simulink model "Vehicle_Model_2Track_OLD"  (R2022b)
settings: Solver=ode2  StartTime=0  StopTime=Tf  FixedStep=Ts  EnableMultiTasking=on
model workspace (MAT data in the model file):
  aKalman = Simulink.Parameter
  aKalman.DataType = 'auto'
  aKalman.Complexity = 'real'
  aKalman.Dimensions = [0 0]
  slipEnabler = Simulink.Parameter
  slipEnabler.DataType = 'auto'
  slipEnabler.Complexity = 'real'
  slipEnabler.Dimensions = [0 0]
values from neighbouring files (symbols this model uses):
  flg = 1    [mainVehicleModel_2Track.m]
  slope = 0.5    [mainVehicleModel_2Track.m]
  steer_des = 10    [mainVehicleModel_2Track.m]
  V_des = 50/3.6    (= 13.8888888889)    [mainVehicleModel_2Track.m]
  X0 = loadInitialConditions(V0)    [mainVehicleModel_2Track.m]
undefined symbols (not defined in the file or in its folder): DiscIntNeverNeededParam
libraries: simulink_extras x12, simulink x2, slpidlib x1
settings Model: Creator=Edoardo  LastModifiedBy=giorg
settings SolverCC: AlgebraicLoopSolver=TrustRegion
settings DataIOCC: LimitDataPoints=on  SaveFormat=StructureWithTime
settings OptimizationCC: BlockReduction=off  DefaultParameterBehavior=Inlined  BufferReuse=off  PassReuseOutputArgsAs=Individual arguments  MaxStackSize=64  EfficientTunableParamExpr=on
settings DebuggingCC: ReadBeforeWriteMsg=DisableAll  WriteAfterWriteMsg=DisableAll  WriteAfterReadMsg=DisableAll  AlgebraicLoopMsg=none  MultiTaskDSMMsg=none  ParameterTunabilityLossMsg=error  PregeneratedLibrarySubsystemCodeDiagnostic=none  SFUnexpectedBacktrackingDiag=warning  SFNoUnconditionalDefaultTransitionDiag=warning  SFExecutionAtInitializationDiag=none  ArithmeticOperatorsInVariantConditions=warning
settings HardwareCC: ProdBitPerInt=16  ProdBitPerPointer=16  ProdBitPerSizeT=16  ProdBitPerPtrDiffT=16  ProdLargestAtomicFloat=None  ProdWordSize=16  ProdHWDeviceType=STMicroelectronics->ST10/Super10
settings ModelReferenceCC: UpdateModelReferenceTargets=IfOutOfDate  EnableRefExpFcnMdlSchedulingChecks=on  PropagateSignalLabelsOutOfModel=off
settings SFSimCC: SFSimEcho=off  SimUseLocalCustomCode=off  MATLABDynamicMemAlloc=off  CustomCodeUndefinedFunction=UseInterfaceOnly
settings RTWCC: Description=Embedded Coder  SystemTargetFile=ert.tlc  TemplateMakefile=ert_default_tmf  GenerateReport=on  RetainRTWFile=on  RTWUseLocalCustomCode=off  Toolchain=GNU Tools for ARM Embedded Processors  BuildConfiguration=Faster Runs  IncludeHyperlinkInReport=on  LaunchReport=on  GenerateTraceInfo=on  GenerateTraceReport=on  GenerateTraceReportSl=on  GenerateTraceReportSf=on  GenerateTraceReportEml=on  DLArmComputeVersion=19.05
settings CodeAppCC: ForceParamTrailComments=on  IgnoreCustomStorageClasses=off  OperatorAnnotations=on  SimulinkDataObjDesc=on  SFDataObjDesc=on  InsertBlockDesc=on
settings ERTTargetCC: CodeReplacementLibrary=ARM Cortex-M (Optimized)  SupportVariableSizeSignals=on  RootIOFormat=Structure reference  ERTCustomFileTemplate=example_file_process.tlc
settings ConfigComp: CovMetricSettings=dw  CovSaveCumulativeToWorkspaceVar=on  CovSaveSingleToWorkspaceVar=on  CovExternalEMLEnable=off
settings ExplorerConfigSet: SimMechanicsOpenEditorOnUpdate=off

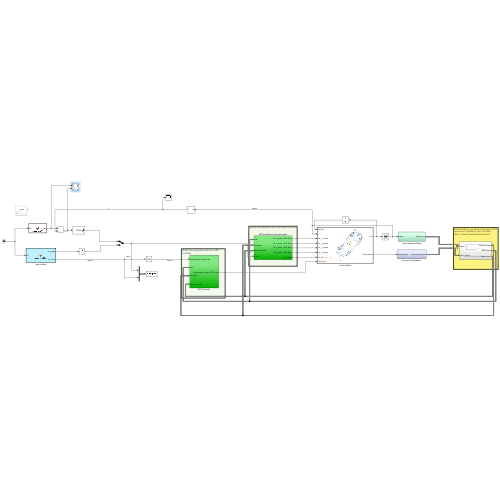
[thumbnail: Simulink's stored preview of the top-level diagram]
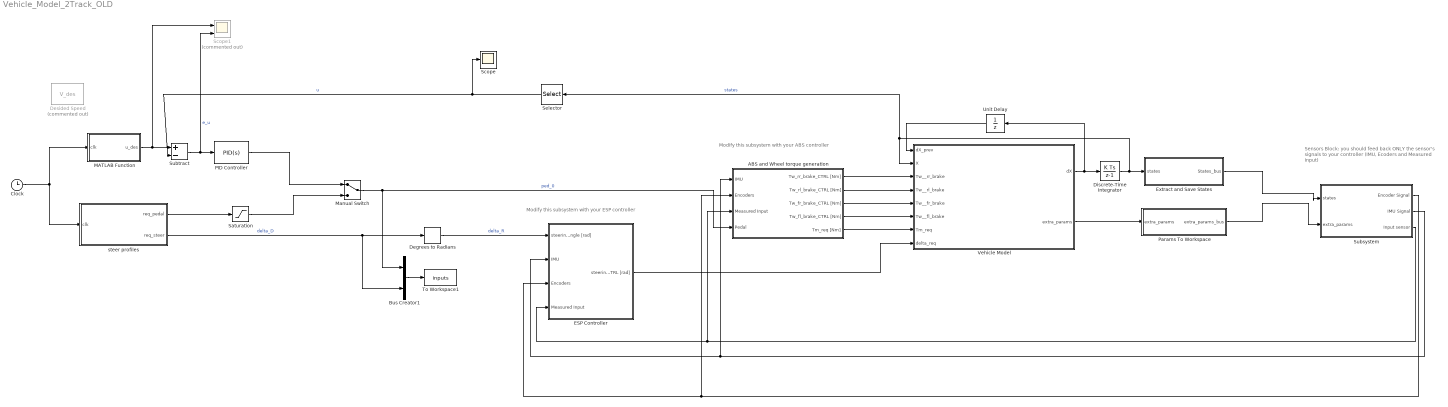
== system Vehicle_Model_2Track_OLD ==
  note: Modify this subsystem with your ESP
      | controller
  note: Modify this subsystem with your ABS controller
  note: Sensors Block: you should feed back ONLY
      | the sensor's signals to your controller
      | (IMU, Ecoders and Measured Input)
  ABS and Wheel torque generation : Subsystem
  Bus Creator1 : BusCreator  Inputs=2
  Clock : Clock
  Degrees to Radians : simulink_extras/Transformations/Degrees to Radians
  Desided Speed : Constant  Commented=on  Value=V_des
  Discrete-Time Integrator : DiscreteIntegrator  gainval=1  InitialCondition=X0  SampleTime=-1  ICPrevOutput=DiscIntNeverNeededParam  ICPrevScaledInput=DiscIntNeverNeededParam
  ESP Controller : Subsystem
  Extract and Save States : Subsystem
  MATLAB Function : MATLAB Function  TreatAsAtomicUnit=on
  Manual Switch : ManualSwitch
  PID Controller : slpidlib/PID Controller  Controller=PID  Form=Parallel  TimeDomain=Continuous-time  UseExternalTs=off  SampleTime=-1  IntegratorMethod=Forward Euler  FilterMethod=Forward Euler  ControllerParametersSource=internal  P=0.0436462066049939  I=0.0175035310088279  UseKiTs=off  D=-0.00909870879334459  N=2  UseFilter=on  TunerSelectOption=Transfer Function Based (PID Tuner App)  InitialConditionSource=internal  InitialConditionForIntegrator=0  InitialConditionForFilter=0  DifferentiatorICPrevScaledInput=0  ExternalReset=none  TrackingMode=off  Kt=1  LimitOutput=on  SatLimitsSource=internal  UpperSaturationLimit=1  LowerSaturationLimit=-1  LinearizeAsGain=on  AntiWindupMode=none  Kb=1  LimitIntegrator=off  UpperIntegratorSaturationLimit=inf  LowerIntegratorSaturationLimit=-inf  POutMin=[]  POutMax=[]  IOutMin=[]  IOutMax=[]  DOutMin=[]  DOutMax=[]  NOutMin=[]  NOutMax=[]  SumOutMin=[]  SumOutMax=[]  SaturationOutMin=[]  SaturationOutMax=[]  PParamMin=[]  PParamMax=[]  IParamMin=[]  IParamMax=[]  DParamMin=[]  DParamMax=[]  NParamMin=[]  NParamMax=[]  KbParamMin=[]  KbParamMax=[]  KtParamMin=[]  KtParamMax=[]  KbOutMin=[]  KbOutMax=[]  KtOutMin=[]  KtOutMax=[]  IntegratorOutMin=[]  IntegratorOutMax=[]  FilterOutMin=[]  FilterOutMax=[]  SumI1OutMin=[]  SumI1OutMax=[]  SumI2OutMin=[]  SumI2OutMax=[]  SumI3OutMin=[]  SumI3OutMax=[]  SumI4OutMin=[]  SumI4OutMax=[]  SumDOutMin=[]  SumDOutMax=[]  DifferentiatorOutMin=[]  DifferentiatorOutMax=[]  FilterDiffOutCoefMin=[]  FilterDiffOutCoefMax=[]  ReciprocalOutMin=[]  ReciprocalOutMax=[]  SumDenOutMin=[]  SumDenOutMax=[]  SumNumOutMin=[]  SumNumOutMax=[]  DivideOutMin=[]  DivideOutMax=[]  UdiffTsProdOutMin=[]  UdiffTsProdOutMax=[]  NTsProdOutMin=[]  NTsProdOutMax=[]  UintegralTsProdOutMin=[]  UintegralTsProdOutMax=[]  UngainTsProdOutMin=[]  UngainTsProdOutMax=[]  ClampingZeroOutDataTypeStr=Inherit: Inherit via back propagation  ClampingZeroOutMin=[]  ClampingZeroOutMax=[]  FilterDenConstantOutDataTypeStr=Inherit: Inherit via back propagation  FilterDenConstantOutMin=[]  FilterDenConstantOutMax=[]  PCopyOutDataTypeStr=Inherit: Inherit via back propagation  PCopyOutMin=[]  PCopyOutMax=[]  NCopyOutDataTypeStr=Inherit: Inherit via back propagation  NCopyOutMin=[]  NCopyOutMax=[]  IntegratorContinuousStateAttributes=''  IntegratorStateMustResolveToSignalObject=off  IntegratorRTWStateStorageClass=Auto  FilterContinuousStateAttributes=''  FilterStateMustResolveToSignalObject=off  FilterRTWStateStorageClass=Auto  ParallelPVariant=InternalParameters  IdealPVariant=Disabled  IVariant=InternalParameters  DVariant=InternalParameters  IntegratorVariant=Continuous  SatVariant=Enabled  AWVariant=Passthrough  PCopyVariant=Disabled  TRVariant=Disabled  FdbkBlocksVariant=Forward  IdealPFdbkVariant=Disabled  SatFdbkVariant=Disabled  DerivativeFilterVariant=ContFilter  NVariant=InternalParameters  NCopyVariant=Disabled  FilterICVariant=InternalICsFilter  IntegratorICVariant=InternalICs  ExternalResetVariant=Disabled  TRSumVariant=Passthrough  SumFdbkVariant=Disabled  SumVariant=Sum_PID  TsampFilterVariant=InternalTs  TsampNgainVariant=Passthrough  TsampIntegralVariant=Passthrough  ExternalSaturationOutDataTypeStr=Inherit: Same as second input
  Params To Workspace : Subsystem
  Saturation : Saturate  UpperLimit=1  LowerLimit=-1
  Scope : Scope
  Scope1 : Scope  Commented=on  NumInputPorts=2
  Selector : Selector  InputPortWidth=23  IndexOptions=Index vector (dialog)  Indices=[4]  OutputSizes=1
  Subsystem : Subsystem
  Subtract : Sum  Inputs=+-
  To Workspace1 : ToWorkspace  VariableName=inputs  SaveFormat=Timeseries  SampleTime=-1
  Unit Delay : UnitDelay  InitialCondition=zeros(size(X0))  SampleTime=-1  HasFrameUpgradeWarning=on
  Vehicle Model : MATLAB Function  TreatAsAtomicUnit=on
  steer profiles : MATLAB Function  TreatAsAtomicUnit=on
  wires:
  Vehicle Model/2(extra_params) -> Params To Workspace/1(extra_params)
  Discrete-Time Integrator/1 -> Extract and Save States/1(states), Selector/1, Vehicle Model/2(X)  "states"
  Vehicle Model/1(dX) -> Unit Delay/1, Discrete-Time Integrator/1
  Bus Creator1/1 -> To Workspace1/1
  steer profiles/2(req_steer) -> Bus Creator1/2, Degrees to Radians/1  "delta_D"
  Unit Delay/1 -> Vehicle Model/1(dX_prev)
  ESP Controller/1(steeringWheel_angle_CTRL [rad]) -> Vehicle Model/8(delta_req)
  Degrees to Radians/1 -> ESP Controller/1(steeringWheel_angle [rad])  "delta_R"
  ABS and Wheel torque generation/1(Tw_rr_brake_CTRL [Nm]) -> Vehicle Model/3(Tw__rr_brake)
  ABS and Wheel torque generation/2(Tw_rl_brake_CTRL [Nm]) -> Vehicle Model/4(Tw__rl_brake)
  ABS and Wheel torque generation/3(Tw_fr_brake_CTRL [Nm]) -> Vehicle Model/5(Tw__fr_brake)
  ABS and Wheel torque generation/4(Tw_fl_brake_CTRL [Nm]) -> Vehicle Model/6(Tw__fl_brake)
  ABS and Wheel torque generation/5(Tm_req [Nm]) -> Vehicle Model/7(Tm_req)
  Extract and Save States/1(States_bus) -> Subsystem/1(states)
  Params To Workspace/1(extra_params_bus) -> Subsystem/2(extra_params)
  Subsystem/1(Encoder Signal) -> ESP Controller/3(Encoders), ABS and Wheel torque generation/2(Encoders)
  Subsystem/2(IMU Signal) -> ESP Controller/2(IMU), ABS and Wheel torque generation/1(IMU)
  Subsystem/3(Input sensor) -> ABS and Wheel torque generation/3(Measured Input), ESP Controller/4(Measured Input)
  Selector/1 -> Scope/1, Subtract/2  "u"
  Subtract/1 -> Scope1/2, PID Controller/1  "e_u"
  steer profiles/1(req_pedal) -> Saturation/1
  MATLAB Function/1(u_des) -> Scope1/1, Subtract/1
  Saturation/1 -> Manual Switch/2
  PID Controller/1 -> Manual Switch/1
  Manual Switch/1 -> Bus Creator1/1, ABS and Wheel torque generation/4(Pedal)  "ped_0"
  Clock/1 -> steer profiles/1(clk), MATLAB Function/1(clk)

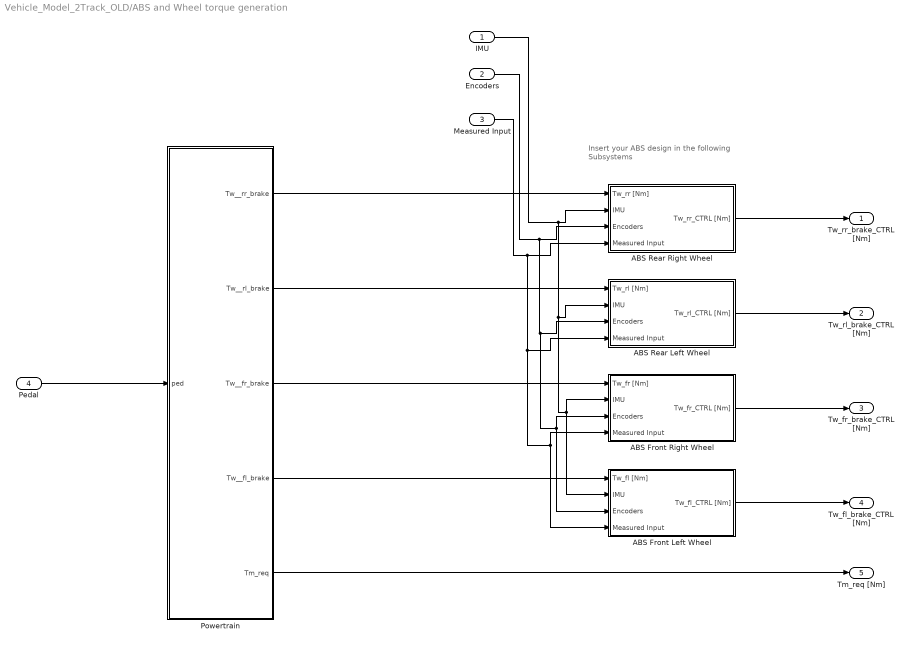
== system Vehicle_Model_2Track_OLD/ABS and Wheel torque generation ==
  note: Insert your ABS design in the
      | following Subsystems
  IMU : Inport
  Encoders : Inport  Port=2
  Measured Input : Inport  Port=3
  Pedal : Inport  Port=4
  ABS Front Left Wheel : Subsystem
  ABS Front Right Wheel : Subsystem
  ABS Rear Left Wheel : Subsystem
  ABS Rear Right Wheel : Subsystem
  Powertrain : MATLAB Function  TreatAsAtomicUnit=on
  Tw_rr_brake_CTRL [Nm] : Outport  VectorParamsAs1DForOutWhenUnconnected=off
  Tw_rl_brake_CTRL [Nm] : Outport  Port=2  VectorParamsAs1DForOutWhenUnconnected=off
  Tw_fr_brake_CTRL [Nm] : Outport  Port=3  VectorParamsAs1DForOutWhenUnconnected=off
  Tw_fl_brake_CTRL [Nm] : Outport  Port=4  VectorParamsAs1DForOutWhenUnconnected=off
  Tm_req [Nm] : Outport  Port=5  VectorParamsAs1DForOutWhenUnconnected=off
  wires:
  Measured Input/1 -> ABS Front Left Wheel/4(Measured Input), ABS Front Right Wheel/4(Measured Input), ABS Rear Left Wheel/4(Measured Input), ABS Rear Right Wheel/4(Measured Input)
  Encoders/1 -> ABS Rear Right Wheel/3(Encoders), ABS Front Right Wheel/3(Encoders), ABS Front Left Wheel/3(Encoders), ABS Rear Left Wheel/3(Encoders)
  IMU/1 -> ABS Rear Left Wheel/2(IMU), ABS Front Left Wheel/2(IMU), ABS Front Right Wheel/2(IMU), ABS Rear Right Wheel/2(IMU)
  Pedal/1 -> Powertrain/1(ped)
  ABS Front Left Wheel/1(Tw_fl_CTRL [Nm]) -> Tw_fl_brake_CTRL [Nm]/1
  ABS Front Right Wheel/1(Tw_fr_CTRL [Nm]) -> Tw_fr_brake_CTRL [Nm]/1
  ABS Rear Left Wheel/1(Tw_rl_CTRL [Nm]) -> Tw_rl_brake_CTRL [Nm]/1
  ABS Rear Right Wheel/1(Tw_rr_CTRL [Nm]) -> Tw_rr_brake_CTRL [Nm]/1
  Powertrain/5(Tm_req) -> Tm_req [Nm]/1
  Powertrain/1(Tw__rr_brake) -> ABS Rear Right Wheel/1(Tw_rr [Nm])
  Powertrain/2(Tw__rl_brake) -> ABS Rear Left Wheel/1(Tw_rl [Nm])
  Powertrain/3(Tw__fr_brake) -> ABS Front Right Wheel/1(Tw_fr [Nm])
  Powertrain/4(Tw__fl_brake) -> ABS Front Left Wheel/1(Tw_fl [Nm])

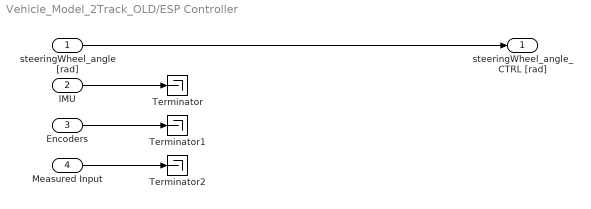
== system Vehicle_Model_2Track_OLD/ESP Controller ==
  steeringWheel_angle [rad] : Inport
  IMU : Inport  Port=2
  Encoders : Inport  Port=3
  Measured Input : Inport  Port=4
  Terminator : Terminator
  Terminator1 : Terminator
  Terminator2 : Terminator
  steeringWheel_angle_CTRL [rad] : Outport  VectorParamsAs1DForOutWhenUnconnected=off
  wires:
  steeringWheel_angle [rad]/1 -> steeringWheel_angle_CTRL [rad]/1
  IMU/1 -> Terminator/1
  Encoders/1 -> Terminator1/1
  Measured Input/1 -> Terminator2/1

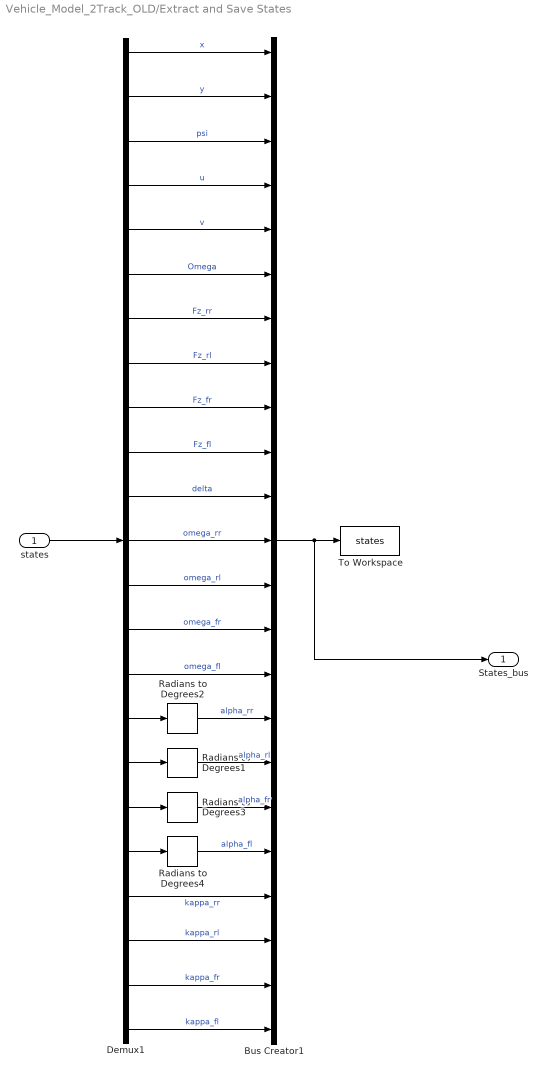
== system Vehicle_Model_2Track_OLD/Extract and Save States ==
  states : Inport
  Bus Creator1 : BusCreator  Inputs=23
  Demux1 : Demux  Outputs=23
  Radians to Degrees{1..4} (4 alike) : simulink_extras/Transformations/Radians to Degrees
  To Workspace : ToWorkspace  VariableName=states  SaveFormat=Timeseries  SampleTime=-1
  States_bus : Outport
  wires:
  Demux1/13 -> Bus Creator1/13  "omega_rl"
  Demux1/8 -> Bus Creator1/8  "Fz_rl"
  Demux1/23 -> Bus Creator1/23  "kappa_fl"
  Demux1/19 -> Radians to Degrees4/1
  states/1 -> Demux1/1
  Demux1/14 -> Bus Creator1/14  "omega_fr"
  Demux1/7 -> Bus Creator1/7  "Fz_rr"
  Demux1/15 -> Bus Creator1/15  "omega_fl"
  Demux1/3 -> Bus Creator1/3  "psi"
  Demux1/22 -> Bus Creator1/22  "kappa_fr"
  Demux1/4 -> Bus Creator1/4  "u"
  Demux1/6 -> Bus Creator1/6  "Omega"
  Demux1/11 -> Bus Creator1/11  "delta"
  Demux1/5 -> Bus Creator1/5  "v"
  Demux1/9 -> Bus Creator1/9  "Fz_fr"
  Demux1/21 -> Bus Creator1/21  "kappa_rl"
  Demux1/12 -> Bus Creator1/12  "omega_rr"
  Demux1/17 -> Radians to Degrees1/1
  Demux1/2 -> Bus Creator1/2  "y"
  Demux1/20 -> Bus Creator1/20  "kappa_rr"
  Demux1/10 -> Bus Creator1/10  "Fz_fl"
  Demux1/18 -> Radians to Degrees3/1
  Demux1/1 -> Bus Creator1/1  "x"
  Demux1/16 -> Radians to Degrees2/1
  Bus Creator1/1 -> States_bus/1, To Workspace/1
  Radians to Degrees2/1 -> Bus Creator1/16  "alpha_rr"
  Radians to Degrees1/1 -> Bus Creator1/17  "alpha_rl"
  Radians to Degrees3/1 -> Bus Creator1/18  "alpha_fr"
  Radians to Degrees4/1 -> Bus Creator1/19  "alpha_fl"

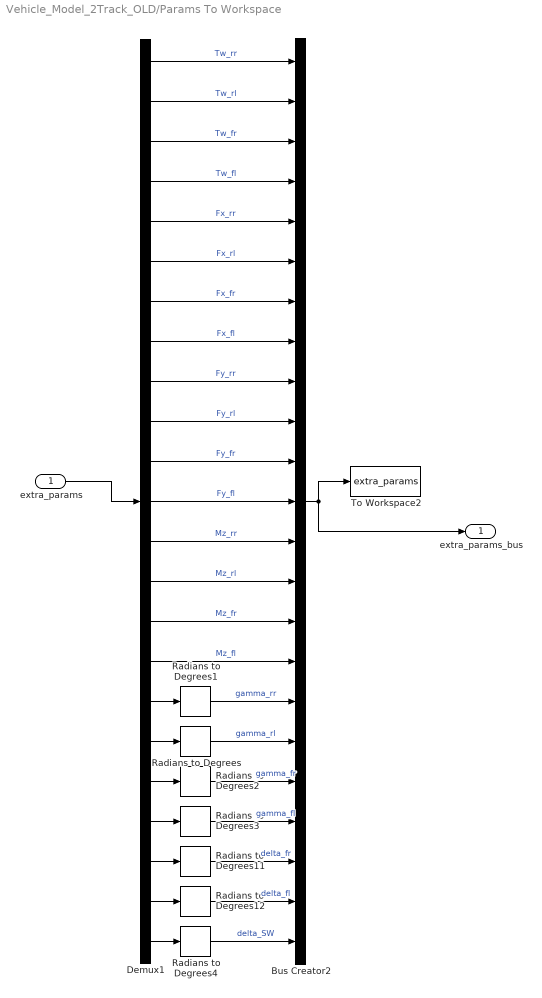
== system Vehicle_Model_2Track_OLD/Params To Workspace ==
  extra_params : Inport
  Bus Creator2 : BusCreator  Inputs=23
  Demux1 : Demux  Outputs=23
  Radians to Degrees{,1..4,11..12} (7 alike) : simulink_extras/Transformations/Radians to Degrees
  To Workspace2 : ToWorkspace  VariableName=extra_params  SaveFormat=Timeseries  SampleTime=-1
  extra_params_bus : Outport
  wires:
  Demux1/17 -> Radians to Degrees1/1
  Demux1/3 -> Bus Creator2/3  "Tw_fr"
  Radians to Degrees3/1 -> Bus Creator2/20  "gamma_fl"
  Demux1/16 -> Bus Creator2/16  "Mz_fl"
  Radians to Degrees1/1 -> Bus Creator2/17  "gamma_rr"
  Radians to Degrees11/1 -> Bus Creator2/21  "delta_fr"
  Demux1/14 -> Bus Creator2/14  "Mz_rl"
  Demux1/4 -> Bus Creator2/4  "Tw_fl"
  Demux1/6 -> Bus Creator2/6  "Fx_rl"
  Demux1/8 -> Bus Creator2/8  "Fx_fl"
  Demux1/13 -> Bus Creator2/13  "Mz_rr"
  Demux1/7 -> Bus Creator2/7  "Fx_fr"
  Demux1/5 -> Bus Creator2/5  "Fx_rr"
  Demux1/9 -> Bus Creator2/9  "Fy_rr"
  Demux1/11 -> Bus Creator2/11  "Fy_fr"
  Demux1/15 -> Bus Creator2/15  "Mz_fr"
  Demux1/10 -> Bus Creator2/10  "Fy_rl"
  Radians to Degrees12/1 -> Bus Creator2/22  "delta_fl"
  Radians to Degrees2/1 -> Bus Creator2/19  "gamma_fr"
  extra_params/1 -> Demux1/1
  Demux1/12 -> Bus Creator2/12  "Fy_fl"
  Bus Creator2/1 -> To Workspace2/1, extra_params_bus/1
  Demux1/1 -> Bus Creator2/1  "Tw_rr"
  Demux1/2 -> Bus Creator2/2  "Tw_rl"
  Radians to Degrees/1 -> Bus Creator2/18  "gamma_rl"
  Demux1/18 -> Radians to Degrees/1
  Demux1/19 -> Radians to Degrees2/1
  Demux1/20 -> Radians to Degrees3/1
  Demux1/21 -> Radians to Degrees11/1
  Demux1/22 -> Radians to Degrees12/1
  Demux1/23 -> Radians to Degrees4/1
  Radians to Degrees4/1 -> Bus Creator2/23  "delta_SW"

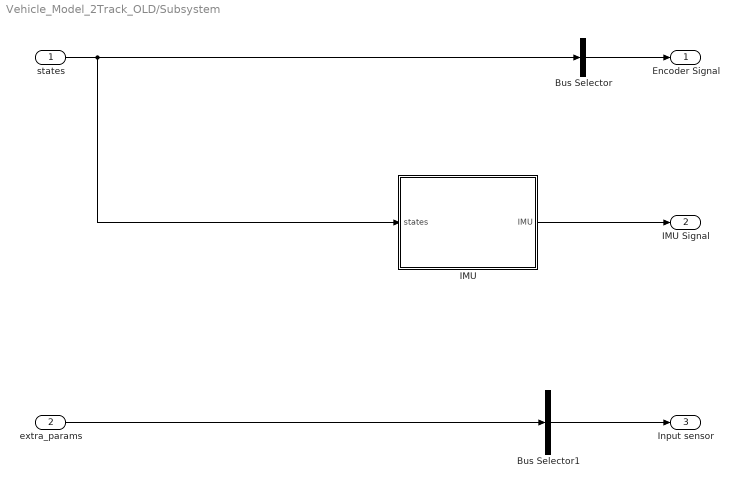
== system Vehicle_Model_2Track_OLD/Subsystem ==
  states : Inport
  extra_params : Inport  Port=2
  Bus Selector : BusSelector  OutputSignals=omega_rr,omega_rl,omega_fr,omega_fl  OutputAsBus=on
  Bus Selector1 : BusSelector  OutputSignals=delta_SW,Tw_rr,Tw_rl,Tw_fr,Tw_fl  OutputAsBus=on
  IMU : Subsystem
  Encoder Signal : Outport  VectorParamsAs1DForOutWhenUnconnected=off
  IMU Signal : Outport  Port=2  VectorParamsAs1DForOutWhenUnconnected=off
  Input sensor : Outport  Port=3  VectorParamsAs1DForOutWhenUnconnected=off
  wires:
  states/1 -> IMU/1(states), Bus Selector/1
  Bus Selector/1 -> Encoder Signal/1
  IMU/1(IMU) -> IMU Signal/1
  extra_params/1 -> Bus Selector1/1
  Bus Selector1/1 -> Input sensor/1

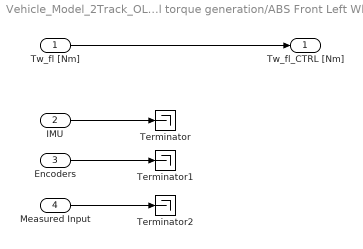
== system Vehicle_Model_2Track_OLD/ABS and Wheel torque generation/ABS Front Left Wheel ==
  Tw_fl [Nm] : Inport
  IMU : Inport  Port=2
  Encoders : Inport  Port=3
  Measured Input : Inport  Port=4
  Terminator : Terminator
  Terminator1 : Terminator
  Terminator2 : Terminator
  Tw_fl_CTRL [Nm] : Outport  VectorParamsAs1DForOutWhenUnconnected=off
  wires:
  Encoders/1 -> Terminator1/1
  Measured Input/1 -> Terminator2/1
  IMU/1 -> Terminator/1
  Tw_fl [Nm]/1 -> Tw_fl_CTRL [Nm]/1

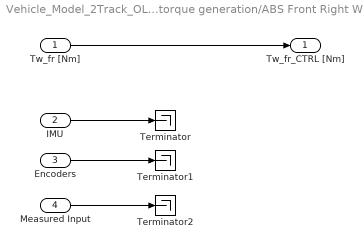
== system Vehicle_Model_2Track_OLD/ABS and Wheel torque generation/ABS Front Right Wheel ==
  Tw_fr [Nm] : Inport
  IMU : Inport  Port=2
  Encoders : Inport  Port=3
  Measured Input : Inport  Port=4
  Terminator : Terminator
  Terminator1 : Terminator
  Terminator2 : Terminator
  Tw_fr_CTRL [Nm] : Outport  VectorParamsAs1DForOutWhenUnconnected=off
  wires:
  Tw_fr [Nm]/1 -> Tw_fr_CTRL [Nm]/1
  IMU/1 -> Terminator/1
  Measured Input/1 -> Terminator2/1
  Encoders/1 -> Terminator1/1

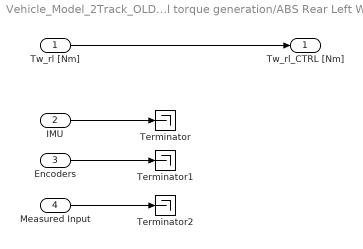
== system Vehicle_Model_2Track_OLD/ABS and Wheel torque generation/ABS Rear Left Wheel ==
  Tw_rl [Nm] : Inport
  IMU : Inport  Port=2
  Encoders : Inport  Port=3
  Measured Input : Inport  Port=4
  Terminator : Terminator
  Terminator1 : Terminator
  Terminator2 : Terminator
  Tw_rl_CTRL [Nm] : Outport  VectorParamsAs1DForOutWhenUnconnected=off
  wires:
  Encoders/1 -> Terminator1/1
  Measured Input/1 -> Terminator2/1
  IMU/1 -> Terminator/1
  Tw_rl [Nm]/1 -> Tw_rl_CTRL [Nm]/1

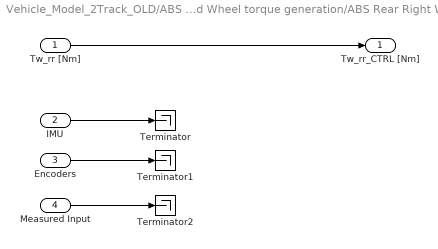
== system Vehicle_Model_2Track_OLD/ABS and Wheel torque generation/ABS Rear Right Wheel ==
  Tw_rr [Nm] : Inport
  IMU : Inport  Port=2
  Encoders : Inport  Port=3
  Measured Input : Inport  Port=4
  Terminator : Terminator
  Terminator1 : Terminator
  Terminator2 : Terminator
  Tw_rr_CTRL [Nm] : Outport  VectorParamsAs1DForOutWhenUnconnected=off
  wires:
  Tw_rr [Nm]/1 -> Tw_rr_CTRL [Nm]/1
  IMU/1 -> Terminator/1
  Measured Input/1 -> Terminator2/1
  Encoders/1 -> Terminator1/1

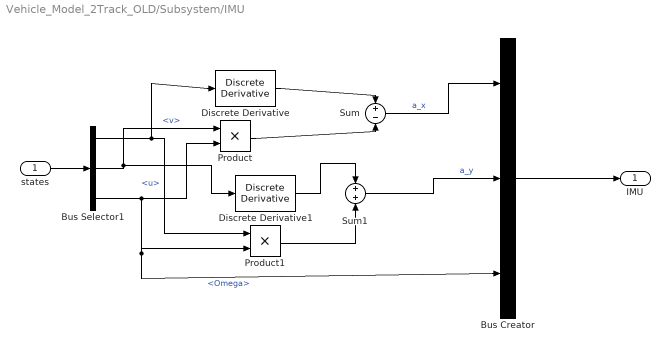
== system Vehicle_Model_2Track_OLD/Subsystem/IMU ==
  states : Inport
  Bus Creator : BusCreator  Inputs=3
  Bus Selector1 : BusSelector  OutputSignals=u,v,Omega
  Discrete Derivative : simulink/Discrete/Discrete Derivative  gainval=1.0  ICPrevScaledInput=0.0  OutMin=[]  OutMax=[]  OutDataType=fixdt(1, 16)  OutScaling=2^-10  DoSatur=off
  Discrete Derivative1 : simulink/Discrete/Discrete Derivative  gainval=1.0  ICPrevScaledInput=0.0  OutMin=[]  OutMax=[]  OutDataType=fixdt(1, 16)  OutScaling=2^-10  DoSatur=off
  Product : Product
  Product1 : Product
  Sum : Sum  Inputs=+-
  Sum1 : Sum
  IMU : Outport
  wires:
  states/1 -> Bus Selector1/1
  Bus Selector1/1 -> Product1/1, Discrete Derivative/1  "<u>"
  Discrete Derivative/1 -> Sum/1
  Product/1 -> Sum/2
  Bus Selector1/2 -> Discrete Derivative1/1, Product/1  "<v>"
  Bus Selector1/3 -> Product1/2, Bus Creator/3, Product/2  "<Omega>"
  Sum/1 -> Bus Creator/1  "a_x"
  Discrete Derivative1/1 -> Sum1/1
  Product1/1 -> Sum1/2
  Sum1/1 -> Bus Creator/2  "a_y"
  Bus Creator/1 -> IMU/1

== matlab function Vehicle_Model_2Track_OLD/ABS and Wheel torque generation/Powertrain ==
  data: ped input; vehicle_data parameter; Tw__rr_brake output; Tw__rl_brake output; Tw__fr_brake output; Tw__fl_brake output; Tm_req output
function [Tw__rr_brake,Tw__rl_brake,Tw__fr_brake,Tw__fl_brake,Tm_req] = powertrain(ped, vehicle_data)

% ----------------------
% MOTOR MODEL
% ----------------------
% Driving torques at the wheels
Tm_req = posPart(ped)*vehicle_data.motor.maxTorque;
 
% ----------------------
% BRAKE MODEL
% ----------------------
Tb_r_req = -negPart(ped)*vehicle_data.braking.totBrakeTorque*(1-vehicle_data.braking.brakeRatio);
Tb_f_req = -negPart(ped)*vehicle_data.braking.totBrakeTorque*vehicle_data.braking.brakeRatio;


% Rear wheels braking model
Tw__rr_brake = Tb_r_req; 
Tw__rl_brake = Tb_r_req; 
% Front wheels braking model
Tw__fr_brake = Tb_f_req; 
Tw__fl_brake = Tb_f_req; 


end

== matlab function Vehicle_Model_2Track_OLD/steer profiles ==
  data: clk input; req_pedal output; req_steer output; steer_des parameter; flg parameter; slope parameter
function [req_pedal,req_steer] = steer_profiles(clk,steer_des,flg, slope)

    % ----------------------------------------------------------------
    %% Function purpose: compute the desired steer profiles
    % Kept separate in case we want to bypass the PID
    % ----------------------------------------------------------------
    
    % Requested pedal for this time step
    if clk > 1
      req_pedal = 0.1; %-0.8;
    else
      req_pedal = 0; %-0.8;
    end
   
    % Requested steering angle [deg] at the steering wheel for this time step
    if flg == 2   % Steer Ramp
        if clk>1
            req_steer = steer_des + clk*slope;
        else
            req_steer = steer_des;
        end
    elseif flg == 1   % Speed Ramp -> Start steering after 1s moving straight 
        
            req_steer = steer_des;
    
    else
    error('Define Test Flag')
    end
end

== matlab function Vehicle_Model_2Track_OLD/MATLAB Function ==
  data: clk input; u_des output; V_des parameter; slope parameter; flg parameter
function u_des = speed_profile(clk,V_des,slope,flg)
% ------------------------------------------------------
% Function to produce speed profiles in input to the PID
% ------------------------------------------------------
if flg == 1         % Speed Ramp

    if clk>1
        u_des = V_des + clk*slope - slope;
    else
        u_des = V_des; 
    end

elseif flg == 2     % Steer Ramp
   u_des = V_des;
else
    error('Define Test Flag')
end

end

== matlab function Vehicle_Model_2Track_OLD/Vehicle Model ==
  settings: sampleTime=step_size
  data: dX_prev input; X input; Tw__rr_brake input; Tw__rl_brake input; Tw__fr_brake input; Tw__fl_brake input; Tm_req input; dX output; extra_params output; delta_req input; vehicle_data parameter
function [dX,extra_params] = Vehicle_model(dX_prev,X,Tw__rr_brake,Tw__rl_brake,Tw__fr_brake,Tw__fl_brake,Tm_req,delta_req,vehicle_data)

% ----------------------------------------------------------------
%% Double Track Vehicle Model
%  authors: 
%  rev. 1.0 Mattia Piccinini & Gastone Pietro Papini Rosati
%  rev. 2.0 Edoardo Pagot
%  date:
%  rev 1.0:    13/10/2020
%  rev 2.0:    16/05/2022
% ----------------------------------------------------------------


% ----------------------------------------------------------------
%% INPUTS OF THE MODEL
% ----------------------------------------------------------------

% Model inputs are: 
%       - requested wheel torques
%       - requested steering angle at the steering wheel delta_req (in [rad])


% ----------------------------------------------------------------
%% OUTPUTS OF THE MODEL
% ----------------------------------------------------------------

% The outputs of the model are the derivatives of all vehicle states,
% collected in the dX vector, as well as some other useful extra parameters 
% to describe vehicle behavior, saved in the extra_params vector

% Empty output vectors are here initialized 
dX = zeros(23,1);  
extra_params = zeros(23,1);  


% ----------------------------------------------------------------
%% STATES OF THE MODEL
% ----------------------------------------------------------------

x         = X(1);       % [m] x-coord of the vehicle CoM
y         = X(2);       % [m] x-coord of the vehicle CoM
psi       = X(3);       % [rad] yaw angle
u         = X(4);       % [m/s] vehicle longitudinal speed
v         = X(5);       % [m/s] vehicle lateral speed
Omega     = X(6);       % [rad/s] yaw rate
Fz__rr    = X(7);       % [N] vertical force for the rear right wheel
Fz__rl    = X(8);       % [N] vertical force for the rear left wheel
Fz__fr    = X(9);       % [N] vertical force for the front right wheel
Fz__fl    = X(10);      % [N] vertical force for the front left wheel
delta     = X(11);      % [rad] steering angle (at the wheel)
omega__rr = X(12);      % [rad/s] rotational speed rear right wheel
omega__rl = X(13);      % [rad/s] rotational speed rear left wheel 
omega__fr = X(14);      % [rad/s] rotational speed front right wheel 
omega__fl = X(15);      % [rad/s] rotational speed front left wheel 
alpha__rr = X(16);      % [rad] side slip angle rear right wheel
alpha__rl = X(17);      % [rad] side slip angle rear left wheel
alpha__fr = X(18);      % [rad] side slip angle front right wheel
alpha__fl = X(19);      % [rad] side slip angle front left wheel
kappa__rr = X(20);      % [-] longitudinal slip rear right wheel
kappa__rl = X(21);      % [-] longitudinal slip rear left wheel
kappa__fr = X(22);      % [-] longitudinal slip front right wheel
kappa__fl = X(23);      % [-] longitudinal slip front left wheel

% ----------------------------------------------------------------
%% AUXILIARY MODELS
% ----------------------------------------------------------------

% ----------------------
% MOTOR MODEL
% ----------------------
% Driving torques at the wheels
Tw__rr_traction = MotorModel(Tm_req,omega__rr,vehicle_data);
Tw__rl_traction = MotorModel(Tm_req,omega__rl,vehicle_data);

% Rear wheels braking model
Tw__rr_brake = brakeModelRear(Tw__rr_brake,omega__rr,vehicle_data); 
Tw__rl_brake = brakeModelRear(Tw__rl_brake,omega__rl,vehicle_data); 
% Front wheels braking model
Tw__fr_brake = brakeModelFront(Tw__fr_brake,omega__fr,vehicle_data);
Tw__fl_brake = brakeModelFront(Tw__fl_brake,omega__fl,vehicle_data);

% Total Torques
Tw__rr = Tw__rr_brake + Tw__rr_traction;
Tw__rl = Tw__rl_brake + Tw__rl_traction;
Tw__fr = Tw__fr_brake;
Tw__fl = Tw__fl_brake;


% ----------------------
% CAMBER MODEL
% ----------------------
[gamma__rr, gamma__rl, gamma__fr, gamma__fl] = camberModel(vehicle_data);

% ----------------------
% ACKERMANN STEERING MODEL
% ----------------------
% Compute steering angles for front wheels, with perfect Ackerman steering model
[delta__fr, delta__fl] = perfectAcker(delta,vehicle_data);

% ----------------------
% AERODYNAMIC MODEL
% ----------------------
% Aero drag, downforce at rear axle, downforce at front axle
[FAxc, FAz__r, FAz__f] = aeroModel(u,vehicle_data);

% ----------------------
% LONGITUDINAL SLIPS
% ----------------------
% Longitudinal slip model including a correction for low speed 
[kappa__rr_corr,kappa__rl_corr,kappa__fr_corr,kappa__fl_corr] = long_slip_low_speed(u,Omega,kappa__rr,kappa__rl,kappa__fr,kappa__fl,omega__rr,omega__rl,omega__fr,omega__fl,delta__fr,delta__fl,Fz__rr,Fz__rl,Fz__fr,Fz__fl,gamma__rr,gamma__rl,gamma__fr,gamma__fl,vehicle_data);
          
% ----------------------
% TIRE PACEJKA MODEL
% ----------------------
% Ensure symmetric behavior of left and right tires by calculating the
% forces and moments for left tires via a previous change of sign of the
% side slip alpha and the camber gamma
% Side slip sign must be changed since data were fitted with reverse alpha
% sign

% RR
Fx__rr =  MF96_FX(kappa__rr_corr, -alpha__rr, -gamma__rr, Fz__rr, vehicle_data.tyre_data_r);
Fy__rr = -MF96_FY(kappa__rr_corr,  alpha__rr, -gamma__rr, Fz__rr, vehicle_data.tyre_data_r); % mirrored
AM__rr = -MF96_MZ(kappa__rr_corr,  alpha__rr, -gamma__rr, Fz__rr, vehicle_data.tyre_data_r); % mirrored

% RL
Fx__rl = MF96_FX(kappa__rl_corr, -alpha__rl, gamma__rl, Fz__rl, vehicle_data.tyre_data_r);
Fy__rl = MF96_FY(kappa__rl_corr, -alpha__rl, gamma__rl, Fz__rl, vehicle_data.tyre_data_r);
AM__rl = MF96_MZ(kappa__rl_corr, -alpha__rl, gamma__rl, Fz__rl, vehicle_data.tyre_data_r);

%FR
Fx__fr =  MF96_FX(kappa__fr_corr, -alpha__fr, -gamma__fr, Fz__fr, vehicle_data.tyre_data_f);
Fy__fr = -MF96_FY(kappa__fr_corr,  alpha__fr, -gamma__fr, Fz__fr, vehicle_data.tyre_data_f); % mirrored
AM__fr = -MF96_MZ(kappa__fr_corr,  alpha__fr, -gamma__fr, Fz__fr, vehicle_data.tyre_data_f); % mirrored

% FL
Fx__fl = MF96_FX(kappa__fl_corr, -alpha__fl, gamma__fl, Fz__fl, vehicle_data.tyre_data_f);
Fy__fl = MF96_FY(kappa__fl_corr, -alpha__fl, gamma__fl, Fz__fl, vehicle_data.tyre_data_f);
AM__fl = MF96_MZ(kappa__fl_corr, -alpha__fl, gamma__fl, Fz__fl, vehicle_data.tyre_data_f);

% Adapt from "adapted SAE" to "ISO"
% Fy = -Fy
% Mz = -Mz
Fy__rr = -Fy__rr;
Fy__rl = -Fy__rl;
Fy__fr = -Fy__fr;
Fy__fl = -Fy__fl;
AM__rr = -AM__rr;
AM__rl = -AM__rl;
AM__fr = -AM__fr;
AM__fl = -AM__fl;

Mz_tires.rr = AM__rr;  Mz_tires.rl = AM__rl;  Mz_tires.fr = AM__fr;  Mz_tires.fl = AM__fl;

% ----------------------
% VERTICAL TIRE FORCES MODEL
% ----------------------
% Compute vertical tire loads
u_dot = dX_prev(4);
VerticalForces = LoadTransferModel(Omega,u,u_dot,FAz__r,FAz__f,Mz_tires,vehicle_data);
Fz__rr__ss = VerticalForces.Fz_rr_ss;
Fz__rl__ss = VerticalForces.Fz_rl_ss;
Fz__fr__ss = VerticalForces.Fz_fr_ss;
Fz__fl__ss = VerticalForces.Fz_fl_ss;

% ----------------------
% AXLE FORCES
% ----------------------
Fx__r = Fx__rr + Fx__rl;
Fx__f = Fx__fl - sin(delta__fl)*Fy__fl + Fx__fr - sin(delta__fr)*Fy__fr;
Fy__r = Fy__rl + Fy__rr;
Fy__f = sin(delta__fl)*Fx__fl + Fy__fl + sin(delta__fr)*Fx__fr + Fy__fr;
Delta__Fx__r = (Fx__rr-Fx__rl)/2;
Delta__Fx__f = ((Fx__fr - sin(delta__fr)*Fy__fr) - (Fx__fl - sin(delta__fl)*Fy__fl))/2;


% ----------------------
% STEADY STATE SLIPS
% ----------------------
% Longitudinal Slips
[kappa__rr__ss,kappa__rl__ss,kappa__fr__ss,kappa__fl__ss] = steadyStateLongSlips(omega__rr,omega__rl,omega__fr,omega__fl,Omega,u,delta__fr,delta__fl,vehicle_data);
% Lateral Slips
[alpha__rr__ss,alpha__rl__ss,alpha__fr__ss,alpha__fl__ss] = steadyStateLatSlips(Omega,u,v,delta__fr,delta__fl,vehicle_data);


% ----------------------------------------------------------------
%% VEHICLE DATA
% ----------------------------------------------------------------
m      = vehicle_data.vehicle.m;
Lf     = vehicle_data.vehicle.Lf;
Lr     = vehicle_data.vehicle.Lr;
Wf     = vehicle_data.vehicle.Wf;
Wr     = vehicle_data.vehicle.Wr;
izz    = vehicle_data.vehicle.i_zz;
tau__N = vehicle_data.suspension.tau_N;
tau__D = vehicle_data.steering_system.tau_D;
tau__H = vehicle_data.steering_system.tau_H;
ly     = vehicle_data.vehicle.ly;
lx     = vehicle_data.vehicle.lx;
iwa__r = vehicle_data.rear_wheel.iwa_r;
iwa__f = vehicle_data.front_wheel.iwa_f;
Rr     = vehicle_data.rear_wheel.Rr;
Rf     = vehicle_data.front_wheel.Rf;

% ----------------------------------------------------------------
%% VEHICLE MODEL DIFFERENTIAL EQUATIONS
% ----------------------------------------------------------------

% The following system of ODE is imported from Maple symbolic model

% Evolution of vehicle pose
x_dot        = u*cos(psi) - v*sin(psi);
y_dot        = v*cos(psi) + u*sin(psi);
psi_dot      = Omega;
% Newton equations
u_Dot        = (Omega * m * v - FAxc + Fx__f + Fx__r) / m;
v_Dot        = (-Omega * m * u + Fy__f + Fy__r) / m;
% Euler equation
Omega_Dot    = (Lf * Fy__f - Lr * Fy__r + Wf * Delta__Fx__f + Wr * Delta__Fx__r + AM__fl + AM__fr + AM__rl + AM__rr) / izz;
% Vertical loads first order dynamics
Fz_rr_Dot    = (-Fz__rr + Fz__rr__ss) / tau__N;
Fz_rl_Dot    = (-Fz__rl + Fz__rl__ss) / tau__N;
Fz_fr_Dot    = (-Fz__fr + Fz__fr__ss) / tau__N;
Fz_fl_Dot    = (-Fz__fl + Fz__fl__ss) / tau__N;
% Steering wheel first order dynamics
delta_Dot    = (-delta * tau__D + delta_req) / tau__D / tau__H;
% Side slip angle first order dynamics
alpha_rr_Dot = -(alpha__rr - alpha__rr__ss) * abs(u) / ly;
alpha_rl_Dot = -(alpha__rl - alpha__rl__ss) * abs(u) / ly;
alpha_fr_Dot = -(alpha__fr - alpha__fr__ss) * abs(u) / ly;
alpha_fl_Dot = -(alpha__fl - alpha__fl__ss) * abs(u) / ly;
% Longitudinal slip first order dynamics
kappa_rr_Dot = -abs(u) * (kappa__rr - kappa__rr__ss) / lx;
kappa_rl_Dot = -abs(u) * (kappa__rl - kappa__rl__ss) / lx;
kappa_fr_Dot = -abs(u) * (kappa__fr - kappa__fr__ss) / lx;
kappa_fl_Dot = -abs(u) * (kappa__fl - kappa__fl__ss) / lx;
% Wheel spin dynamics
omega_rr_Dot = (-Fx__rr * Rr + Tw__rr) / iwa__r;
omega_rl_Dot = (-Fx__rl * Rr + Tw__rl) / iwa__r;
omega_fr_Dot = (-Fx__fr * Rf + Tw__fr) / iwa__f;
omega_fl_Dot = (-Fx__fl * Rf + Tw__fl) / iwa__f;

% Collect states derivatives in the dX vector
dX(1)  = x_dot;
dX(2)  = y_dot;
dX(3)  = psi_dot;
dX(4)  = u_Dot;
dX(5)  = v_Dot;
dX(6)  = Omega_Dot;
dX(7)  = Fz_rr_Dot;
dX(8)  = Fz_rl_Dot;
dX(9)  = Fz_fr_Dot;
dX(10) = Fz_fl_Dot;
dX(11) = delta_Dot;
dX(12) = omega_rr_Dot;
dX(13) = omega_rl_Dot;
dX(14) = omega_fr_Dot;
dX(15) = omega_fl_Dot;
dX(16) = alpha_rr_Dot;
dX(17) = alpha_rl_Dot;
dX(18) = alpha_fr_Dot;
dX(19) = alpha_fl_Dot;
dX(20) = kappa_rr_Dot;
dX(21) = kappa_rl_Dot;
dX(22) = kappa_fr_Dot;
dX(23) = kappa_fl_Dot;


% ----------------------------------------------------------------
%% SAVE USEFUL EXTRA PARAMETERS
% ----------------------------------------------------------------

extra_params(1)  = Tw__rr;
extra_params(2)  = Tw__rl;
extra_params(3)  = Tw__fr;
extra_params(4)  = Tw__fl;
extra_params(5)  = Fx__rr;
extra_params(6)  = Fx__rl;
extra_params(7)  = Fx__fr;
extra_params(8)  = Fx__fl;
extra_params(9)  = Fy__rr;
extra_params(10) = Fy__rl;
extra_params(11) = Fy__fr;
extra_params(12) = Fy__fl;
extra_params(13) = AM__rr;
extra_params(14) = AM__rl;
extra_params(15) = AM__fr;
extra_params(16) = AM__fl;
extra_params(17) = gamma__rr;
extra_params(18) = gamma__rl;
extra_params(19) = gamma__fr;
extra_params(20) = gamma__fl;
extra_params(21) = delta__fr;
extra_params(22) = delta__fl;
extra_params(23) = delta_req;

end
